simulink model "rand_pumpModel"  (R2017a)
settings: Solver=VariableStepAuto  StartTime=0.0  StopTime=10.0  RelTol=1e-3
undefined symbols (not defined in the file or in its folder): keta
settings Model: Creator=bogdan.tamas  LastModifiedBy=bogdan.tamas

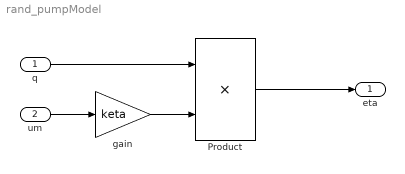
== system rand_pumpModel ==
  "q " : Inport
  um : Inport  Port=2
  Product : Product
  gain : Gain  Gain=keta
  eta : Outport
  wires:
  gain/1 -> Product/2
  Product/1 -> eta/1
  "q "/1 -> Product/1
  um/1 -> gain/1
